simulink model "part6_extracredit_windowstarget_switchingcontrol"  (R2014a)
settings: Solver=ode1  StartTime=0.0  StopTime=1000  FixedStep=0.005  RelTol=1e-3
libraries: c6xlib x2, fricblocks x1
Description:
  | Real-Time Van der Pol Simulation
  | 
  | This demonstration shows a real-time version of the Simulink(R) Van der Pol
  | simulation demo. This model does not need any external signals, so it does
  | not need any data acquisition hardware or driver. This makes the model ideal
  | for first experiments with Real-Time Windows Target(TM), without need to
  | worry about proper I/O hardware configuration.
  | 
  | How to run this demo:
  | 
  |   1. Build the model using Tools -> Real-Time Workshop -> Build Model.
  |   2. Connect to the real-time code using Simulation -> Connect to target.
  |   3. Start the real-time execution using Simulation -> Start real-time code.
settings Model: SimulationMode=external  ExtModeTrigDuration=50000  Creator=Houska  LastModifiedBy=mmroman2
settings DataIOCC: SignalLoggingSaveFormat=ModelDataLogs  SignalLoggingName=logsOut
settings OptimizationCC: ExpressionDepthLimit=2147483647  InitFltsAndDblsToZero=on  EfficientMapNaN2IntZero=off
settings DebuggingCC: UnderspecifiedInitializationDetection=Classic  SignalResolutionControl=TryResolveAllWithWarning  SolverPrmCheckMsg=none  FcnCallInpInsideContextMsg=UseLocalSettings  StateNameClashWarn=warning
settings HardwareCC: ProdIntDivRoundTo=Zero  ProdEndianess=LittleEndian  ProdHWDeviceType=32-bit Real-Time Windows Target
settings RTWCC: SystemTargetFile=rtwin.tlc  TemplateMakefile=rtwin.tmf  Description=Real-Time Windows Target  ProcessScript=rtwin_make_rtw_hook
settings RTWinTargetCC: TargetLibSuffix=_rtwin.lib  TargetPreCompLibLocation=C:\MATLABR2014a\toolbox\rtw\targets\rtwin\lib\win64

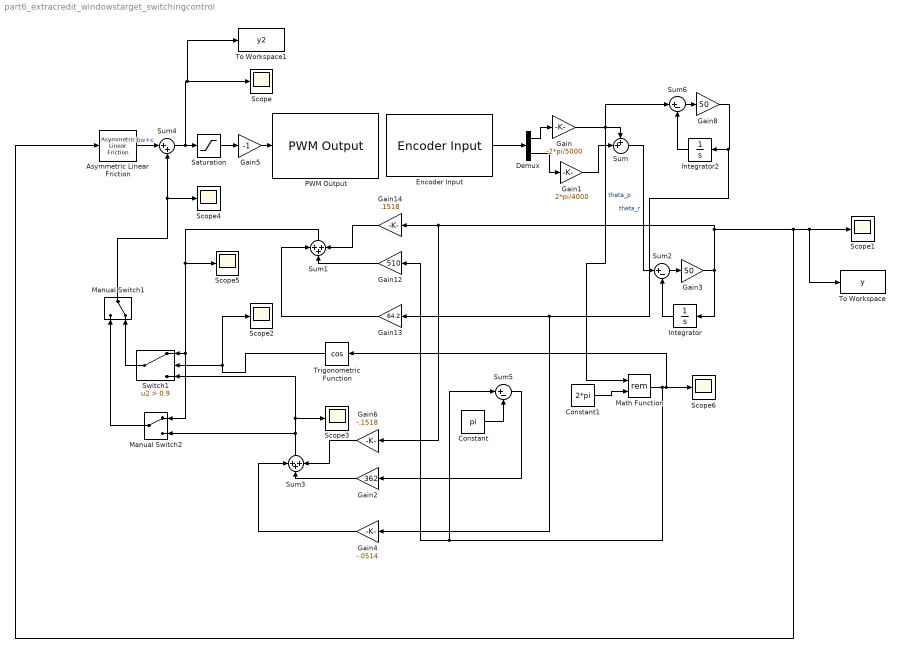
== system part6_extracredit_windowstarget_switchingcontrol ==
  Asymmetric Linear Friction : fricblocks/Asymmetric  Linear Friction  intercept1=.72  intercept2=-.76  slope1=.015  slope2=.016
  Constant : Constant  Value=pi
  Constant1 : Constant  Value=2*pi
  Demux : Demux  Outputs=2
  Encoder Input : c6xlib/Encoder Input  baseAddr=0x378  channels=[0 1]  sampleTime=str2num(get_param(bdroot, 'FixedStep'))
  Gain : Gain  Gain=-2*pi/5000
  Gain1 : Gain  Gain=2*pi/4000
  Gain12 : Gain  Gain=510
  Gain13 : Gain  Gain=64.2
  Gain14 : Gain  Gain=.1518
  Gain2 : Gain  Gain=362
  Gain3 : Gain  Gain=50
  Gain4 : Gain  Gain=-.0514
  Gain5 : Gain  Gain=-1
  Gain6 : Gain  Gain=-.1518
  Gain8 : Gain  Gain=50
  Integrator : Integrator
  Integrator2 : Integrator
  Manual Switch1 : ManualSwitch  CurrentSetting=0
  Manual Switch2 : ManualSwitch
  Math Function : Math  Operator=rem  SaturateOnIntegerOverflow=on
  PWM Output : c6xlib/PWM Output  baseAddr=0x378  channels=0  initialOutputs=0  finalOutputs=0  sampleTime=str2num(get_param(bdroot, 'FixedStep'))
  Saturation : Saturate  UpperLimit=10  LowerLimit=-10
  Scope{,1..6} (7 alike) : Scope
      Scope1 settings: YMin=0  YMax=95
      Scope2 settings: YMin=-0.5  YMax=1  SaveName=ScopeData2
      Scope3 settings: YMin=-0.24  YMax=-0.175  SaveName=ScopeData3
      Scope4 settings: YMin=-0.7  YMax=0.25  SaveName=ScopeData4
      Scope5 settings: YMin=177.5  YMax=186.5  SaveName=ScopeData5
      Scope6 settings: YMin=1.38778e-17  YMax=0.4  SaveName=ScopeData6
  Sum : Sum  Inputs=++|
  Sum1 : Sum  Inputs=+++
  Sum2 : Sum  Inputs=|+-
  Sum3 : Sum  Inputs=+++
  Sum4 : Sum  Inputs=|++
  Sum5 : Sum  Inputs=|+-
  Sum6 : Sum  Inputs=|+-
  Switch1 : Switch  Criteria=u2 > Threshold  Threshold=0.9
  To Workspace : ToWorkspace  VariableName=y  SampleTime=-1
  To Workspace1 : ToWorkspace  VariableName=y2  SampleTime=-1
  Trigonometric Function : Trigonometry  Operator=cos
  wires:
  Demux/2 -> Gain1/1
  Demux/1 -> Gain/1
  Encoder Input/1 -> Demux/1
  Gain1/1 -> Sum/2
  Sum/1 -> Sum2/1  "theta_r"
  Integrator/1 -> Sum2/2
  Sum2/1 -> Gain3/1
  Saturation/1 -> Gain5/1
  Gain5/1 -> PWM Output/1
  Sum4/1 -> To Workspace1/1, Scope/1, Saturation/1
  Integrator2/1 -> Sum6/2
  Sum6/1 -> Gain8/1
  Asymmetric Linear Friction/1 -> Sum4/1  "bw+c"
  Gain14/1 -> Sum1/3
  Gain12/1 -> Sum1/2
  Gain13/1 -> Sum1/1
  Gain/1 -> Sum6/1, Math Function/1, Sum/1  "theta_p"
  Gain3/1 -> Integrator/1, To Workspace/1, Scope1/1, Asymmetric Linear Friction/1, Gain6/1, Gain14/1
  Gain8/1 -> Gain4/1, Gain13/1, Integrator2/1
  Gain6/1 -> Sum3/3
  Gain2/1 -> Sum3/2
  Gain4/1 -> Sum3/1
  Sum5/1 -> Gain2/1
  Constant/1 -> Sum5/2
  Trigonometric Function/1 -> Switch1/2, Scope2/1
  Sum3/1 -> Manual Switch2/2, Scope3/1, Switch1/3
  Sum1/1 -> Scope5/1, Manual Switch2/1, Switch1/1
  Manual Switch1/1 -> Scope4/1, Sum4/2
  Switch1/1 -> Manual Switch1/2
  Manual Switch2/1 -> Manual Switch1/1
  Constant1/1 -> Math Function/2
  Math Function/1 -> Gain12/1, Sum5/1, Trigonometric Function/1, Scope6/1
